simulink model "velocity_feedback"  (Simulink 8.5)
settings: Solver=ode3  StartTime=0.0  StopTime=inf  FixedStep=.002  RelTol=1e-3
undefined symbols (not defined in the file or in its folder): arm_m2jp, bit, CAN_init, enc_per_rev, FT_init, MT_init, sample_time, Standard, VL1_init, VL2_init
libraries: slrtlib x8, simulink x4, slrtsoftinglib x3, xpcutilitieslib x1
settings Model: Creator=Matt Courtney  LastModifiedBy=User
settings SolverCC: EnableConcurrentExecution=on
settings OptimizationCC: BlockReduction=off  BooleanDataType=off  OptimizeBlockIOStorage=off  BufferReuse=off  GlobalBufferReuse=off  ExpressionFolding=off  LocalBlockOutputs=off  InitFltsAndDblsToZero=on
settings DebuggingCC: SolverPrmCheckMsg=warning  FcnCallInpInsideContextMsg=UseLocalSettings  StrictBusMsg=Warning
settings HardwareCC: ProdIntDivRoundTo=Zero  ProdEndianess=LittleEndian  ProdLongLongMode=on  ProdHWDeviceType=Generic->32-bit x86 compatible
settings RTWCC: SystemTargetFile=slrt.tlc  TemplateMakefile=slrt_default_tmf  Description=Simulink Real-Time  RTWCompilerOptimization=on
settings SimulinkRealTimeCC: GeneratePreprocessorConditionals=Disable all  xPCisModelTimeout=off  xPCModelTimeoutSecs=10

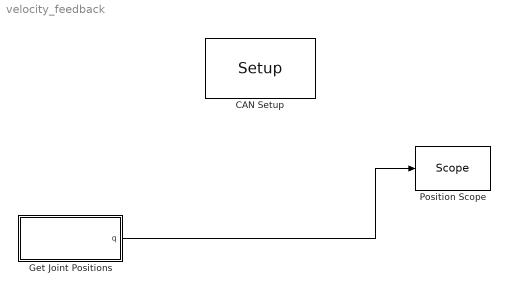
== system velocity_feedback ==
  "CAN Setup " : slrtsoftinglib/CAN-AC2-PCI SJA 1000/Setup   board=1  can1bus=Highspeed (ISO 11898)  can1Baudrate=1 MBaud  can1UserBR=[1,1,4,3]  can2bus=Highspeed (ISO 11898)  can2Baudrate=1 MBaud  can2UserBR=[1,1,4,3]  init=[VL1_init,VL2_init,CAN_init,FT_init,MT_init]  term=[]  bus_off_out=off  bus_off_rec=Off  ioBaseAddress=-1
  Get Joint Positions : Subsystem
  Position Scope : slrtlib/Displays and Logging/Scope   scopeno=5  scopetype=Target  autostart=on  viewmode=Numerical  formatstr=['joint_1 %13.8f rad,joint_2 %13.8f rad,joint_3 %13.8f rad,joint_4 %13.8f rad,joint_5 %13.8f rad,joint_6 %13.8f rad,joint_7 %13.8f rad']  grid=on  ylimits=[0,0]  nosamples=1/(10*sample_time)  noprepostsamples=0  interleave=1  triggermode=FreeRun  triggersignal=1  trigsignalfromport=off  triggerlevel=0.0  triggerslope=Either  triggerscope=1  triggersample=0  filename=data.dat  mode=Lazy  writesize=512  autorestart=off  dynamicfilemode=off  maxwritefilesize=512*1024^2
  wires:
  Get Joint Positions/1(q) -> Position Scope/1

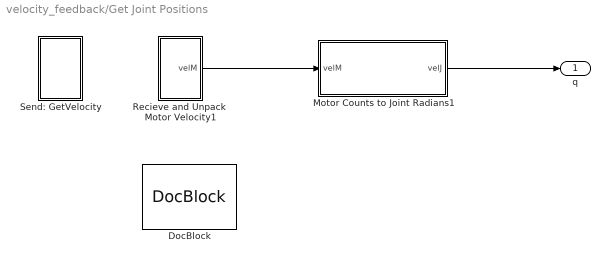
== system velocity_feedback/Get Joint Positions ==
  DocBlock : simulink/Model-Wide Utilities/DocBlock  DocumentType=Text
  Motor Counts to Joint Radians1 : Subsystem
  Recieve and Unpack  Motor Velocity1 : Subsystem
  Send: GetVelocity : Subsystem
  q : Outport
  wires:
  Motor Counts to Joint Radians1/1(velJ) -> q/1
  Recieve and Unpack  Motor Velocity1/1(velM) -> Motor Counts to Joint Radians1/1(velM)

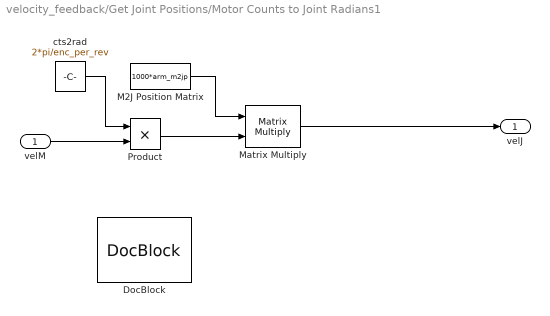
== system velocity_feedback/Get Joint Positions/Motor Counts to Joint Radians1 ==
  velM : Inport
  DocBlock : simulink/Model-Wide Utilities/DocBlock  DocumentType=Text
      content=|
      | Here we do the simple conversion from motor position to joint position,
      | then convert encoder counts to joint radians, then account for the offset
      | in the home position to finally output the joint position in radians. The
      | M2J position matrix can be found in the documentation. Joint 4 has a -18 as
      | opposed to +18 because the motor was reversed at one point during a repair.
      | I believe newer models of the WAM adhere to this -18.
  M2J Position Matrix : Constant  Value=1000*arm_m2jp
  Matrix Multiply : Product  Multiplication=Matrix(*)
  Product : Product  OutMin=[-8192]  OutMax=[8191]  RndMeth=Zero
  cts2rad : Constant  Value=2*pi/enc_per_rev
  velJ : Outport
  wires:
  velM/1 -> Product/2
  Matrix Multiply/1 -> velJ/1
  cts2rad/1 -> Product/1
  M2J Position Matrix/1 -> Matrix Multiply/1
  Product/1 -> Matrix Multiply/2

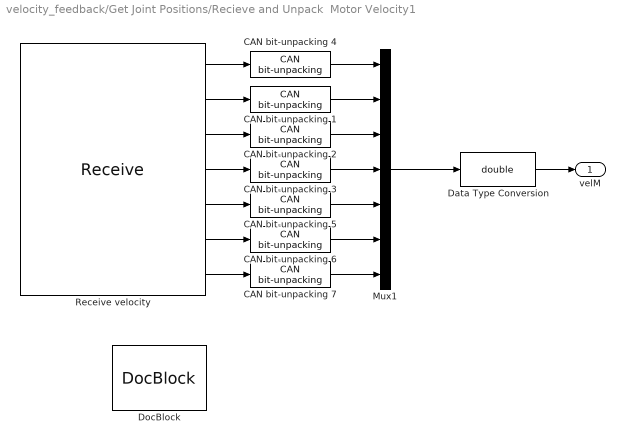
== system velocity_feedback/Get Joint Positions/Recieve and Unpack  Motor Velocity1 ==
  CAN bit-unpacking {1..7} (7 alike) : slrtlib/CAN/Utilities/CAN bit-unpacking   bitpatterns={ [8:15, 16:23, 24:31, 32:39] }  dtypes={ 'int32'}
  Data Type Conversion : DataTypeConversion  OutDataTypeStr=double
  DocBlock : simulink/Model-Wide Utilities/DocBlock  DocumentType=Text
  Mux1 : Mux  Inputs=7
  "Receive velocity " : slrtsoftinglib/CAN-AC2-PCI SJA 1000/Receive   board=1  canPort=CAN 1  range=Standard (11-bit)  ids=[bin2dec('10000100110'),bin2dec('10001000110'),bin2dec('10001100110'),bin2dec('10010000110'),bin2dec('10010100110'),bin2dec('10011000110'),bin2dec('10011100110')]  lengths=0  output=Data  inten=on  ts=sample_time  ididx=[0,1,2,3,5,6,7]
  velM : Outport
  wires:
  Mux1/1 -> Data Type Conversion/1
  "Receive velocity "/1 -> CAN bit-unpacking 4/1
  "Receive velocity "/2 -> CAN bit-unpacking 1/1
  "Receive velocity "/3 -> CAN bit-unpacking 2/1
  "Receive velocity "/4 -> CAN bit-unpacking 3/1
  CAN bit-unpacking 4/1 -> Mux1/1
  CAN bit-unpacking 1/1 -> Mux1/2
  CAN bit-unpacking 2/1 -> Mux1/3
  CAN bit-unpacking 3/1 -> Mux1/4
  Data Type Conversion/1 -> velM/1
  "Receive velocity "/5 -> CAN bit-unpacking 5/1
  "Receive velocity "/6 -> CAN bit-unpacking 6/1
  "Receive velocity "/7 -> CAN bit-unpacking 7/1
  CAN bit-unpacking 5/1 -> Mux1/5
  CAN bit-unpacking 6/1 -> Mux1/6
  CAN bit-unpacking 7/1 -> Mux1/7

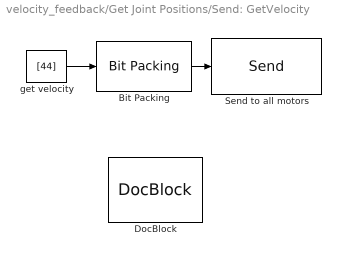
== system velocity_feedback/Get Joint Positions/Send: GetVelocity ==
  Bit Packing : xpcutilitieslib/Bit Packing   MaskBitPatterns={[0:7]}  MaskPackDataType=double  MaskPackDataSize=[1]
  DocBlock : simulink/Model-Wide Utilities/DocBlock  DocumentType=Text
  Send to all motors : slrtsoftinglib/CAN-AC2-PCI SJA 1000/Send   board=1  canPort=CAN 1  range=Standard (11-bit)  ids=1024  sizes=[1]  output=off  ts=sample_time  ididx=[2]
  get velocity : Constant  Value=[44]  OutDataTypeStr=int8
  wires:
  Bit Packing/1 -> Send to all motors/1
  get velocity/1 -> Bit Packing/1
